simulink model "Problem_1"  (R2020a)
settings: Solver=VariableStepAuto  StartTime=0.0  StopTime=10.0  RelTol=1e-3
settings Model: Creator=Saqlain  LastModifiedBy=Saqlain

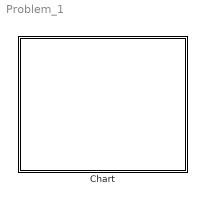
== system Problem_1 ==
  Chart : Stateflow chart  TreatAsAtomicUnit=on

== stateflow chart Problem_1/Chart ==
  state digit1
    state one
      entry:
      p1=1;
    state two
      entry:
      p1=2;
    state zero
      entry:
      p1=0;
    state three
      entry:
      p1=3;
    state four
      entry:
      p1=4;
    digit1.two -> digit1.three : inputclick
    digit1.zero -> digit1.one : inputclick
    digit1.one -> digit1.two : inputclick
    (default) -> digit1.zero
    digit1.four -> digit1.zero : inputclick/{digit2.inc2;}
    digit1.three -> digit1.four : inputclick
  state digit2
    state one
      entry:
      p2=1;
    state two
      entry:
      p2=2;
    state zero
      entry:
      p2=0;
    state three
      entry:
      p2=3;
    state four
      entry:
      p2=4;
    digit2.two -> digit2.three : inc2
    digit2.zero -> digit2.one : inc2
    digit2.one -> digit2.two : inc2
    (default) -> digit2.zero
    digit2.four -> digit2.zero : inc2/{digit3.inc3;}
    digit2.three -> digit2.four : inc2
  events: inc2 local FUNCTION_CALL_EVENT
